simulink model "drive"  (R2017a)
settings: Solver=ode45  StartTime=0.0  StopTime=50  MaxStep=0.1  RelTol=1e-8  AbsTol=1e-7  EnableMultiTasking=on
values from neighbouring files (symbols this model uses):
  dt = -1    [Initdrive.m]
  fd = 4.2    [Initdrive.m]
  initvel = init_speed/3.6    (= 0)    [Initdrive.m]
  M = 1420    [Initdrive.m]    (also in model_setup.m = 400)
  omega = torque_curve(:,1)    [Initdrive.m]
  rad = 0.285    [Initdrive.m]
  throttle = [0  2  2.1  50 ... (first row only)    [Initdrive.m]
  torq = torque_curve(:,2)    [Initdrive.m]
settings Model: ExtModeTrigMode=oneshot  ExtModeArmWhenConnect=off  Creator=ttmcb  LastModifiedBy=ttmcb
settings DataIOCC: SaveFormat=Array  SignalLoggingSaveFormat=ModelDataLogs  SaveOutput=off  SaveTime=off
settings OptimizationCC: BooleanDataType=off  LifeSpan=inf
settings DebuggingCC: SaveWithParameterizedLinksMsg=none  UnderspecifiedInitializationDetection=Classic  MergeDetectMultiDrivingBlocksExec=none  SignalResolutionControl=TryResolveAllWithWarning  MultiTaskDSMMsg=warning  MultiTaskCondExecSysMsg=none  SFUnexpectedBacktrackingDiag=warning  SFNoUnconditionalDefaultTransitionDiag=warning  SFExecutionAtInitializationDiag=none
settings HardwareCC: ProdBitPerPointer=32  ProdBitPerSizeT=32  ProdBitPerPtrDiffT=32  ProdLargestAtomicFloat=None  ProdIntDivRoundTo=Undefined  ProdEndianess=Unspecified  ProdWordSize=32  ProdHWDeviceType=32-bit Generic  TargetUnknown=on
settings ModelReferenceCC: PropagateSignalLabelsOutOfModel=off
settings GRTTargetCC: TargetLangStandard=C89/C90 (ANSI)  GeneratePreprocessorConditionals=Disable all  CombineOutputUpdateFcns=off  GRTInterface=on
settings ConfigComp: CovMetricSettings=dw  CovHtmlReporting=on  CovSaveCumulativeToWorkspaceVar=on  CovSaveSingleToWorkspaceVar=on  CovExternalEMLEnable=off

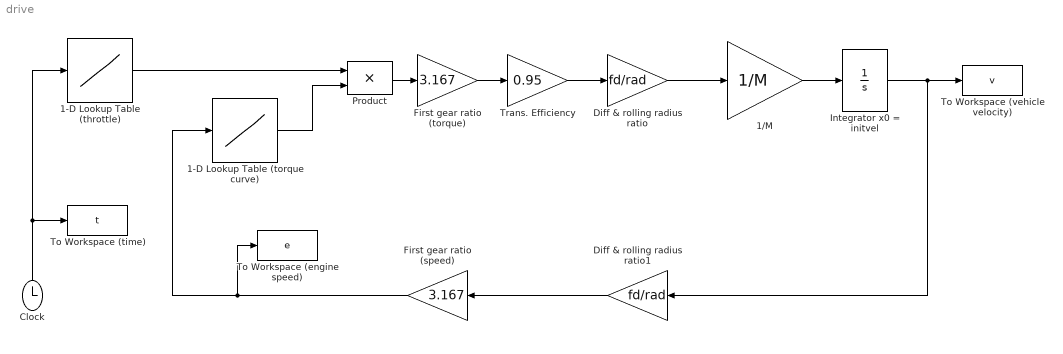
== system drive ==
  1-D Lookup Table (throttle) : Lookup_n-D  NumberOfTableDimensions=1  BreakpointsForDimension1=throttle(1,:)  Table=throttle(2,:)  InternalRulePriority=Speed  RndMeth=Simplest  InputSameDT=on
  1-D Lookup Table (torque curve) : Lookup_n-D  NumberOfTableDimensions=1  BreakpointsForDimension1=omega  Table=torq  InternalRulePriority=Speed  RndMeth=Simplest  InputSameDT=on
  1/M : Gain  Gain=1/M  SaturateOnIntegerOverflow=on  OutDataTypeStr=Inherit: Same as input  ParamDataTypeStr=Inherit: Same as input
  Clock : Clock
  Diff & rolling radius ratio : Gain  Gain=fd/rad  SaturateOnIntegerOverflow=on  OutDataTypeStr=Inherit: Same as input  ParamDataTypeStr=Inherit: Same as input
  Diff & rolling radius ratio1 : Gain  Gain=fd/rad  SaturateOnIntegerOverflow=on  OutDataTypeStr=Inherit: Same as input  ParamDataTypeStr=Inherit: Same as input
  First gear ratio (speed) : Gain  Gain=3.167  SaturateOnIntegerOverflow=on  OutDataTypeStr=Inherit: Same as input  ParamDataTypeStr=Inherit: Same as input
  First gear ratio (torque) : Gain  Gain=3.167  SaturateOnIntegerOverflow=on  OutDataTypeStr=Inherit: Same as input  ParamDataTypeStr=Inherit: Same as input
  Integrator x0 = initvel : Integrator  InitialCondition=initvel  LowerSaturationLimit=0
  Product : Product  SaturateOnIntegerOverflow=on  RndMeth=Zero  InputSameDT=on  OutDataTypeStr=Inherit: Same as first input
  To Workspace (engine speed) : ToWorkspace  VariableName=e  SampleTime=dt
  To Workspace (time) : ToWorkspace  VariableName=t  SampleTime=dt
  To Workspace (vehicle velocity) : ToWorkspace  VariableName=v  SampleTime=dt
  Trans. Efficiency : Gain  Gain=0.95  SaturateOnIntegerOverflow=on  OutDataTypeStr=Inherit: Same as input  ParamDataTypeStr=Inherit: Same as input
  wires:
  Clock/1 -> To Workspace (time)/1, 1-D Lookup Table (throttle)/1
  Diff & rolling radius ratio1/1 -> First gear ratio (speed)/1
  First gear ratio (speed)/1 -> To Workspace (engine speed)/1, 1-D Lookup Table (torque curve)/1
  1-D Lookup Table (throttle)/1 -> Product/1
  1-D Lookup Table (torque curve)/1 -> Product/2
  1/M/1 -> Integrator x0 = initvel/1
  Integrator x0 = initvel/1 -> To Workspace (vehicle velocity)/1, Diff & rolling radius ratio1/1
  Trans. Efficiency/1 -> Diff & rolling radius ratio/1
  Diff & rolling radius ratio/1 -> 1/M/1
  First gear ratio (torque)/1 -> Trans. Efficiency/1
  Product/1 -> First gear ratio (torque)/1
